simulink model "m20212022"  (R2016a)
settings: Solver=VariableStepAuto  StartTime=0.0  StopTime=1  RelTol=1e-3
libraries: simulink x2
settings Model: Creator=witkey721  LastModifiedBy=witkey721

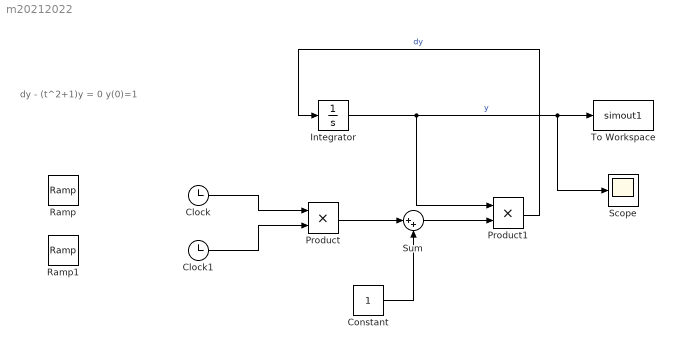
== system m20212022 ==
  note: dy - (t^2+1)y = 0 y(0)=1
  Clock : Clock
  Clock1 : Clock
  Constant : Constant
  Integrator : Integrator  InitialCondition=1
  Product : Product
  Product1 : Product
  Ramp : simulink/Sources/Ramp  slope=1  start=0  X0=0
  Ramp1 : simulink/Sources/Ramp  slope=1  start=0  X0=0
  Scope : Scope
  Sum : Sum  Inputs=|++
  To Workspace : ToWorkspace  VariableName=simout1  SaveFormat=Timeseries  SampleTime=-1
  wires:
  Integrator/1 -> Product1/1, Scope/1, To Workspace/1  "y"
  Product1/1 -> Integrator/1  "dy"
  Product/1 -> Sum/1
  Constant/1 -> Sum/2
  Sum/1 -> Product1/2
  Clock/1 -> Product/1
  Clock1/1 -> Product/2
